simulink model "Subsystem2"  (R2020a)
settings: Solver=VariableStepAuto  StartTime=0.0  StopTime=10.0  RelTol=1e-3
settings Model: Creator=anjal  LastModifiedBy=anjal
settings DataIOCC: SaveOutput=off  SaveTime=off

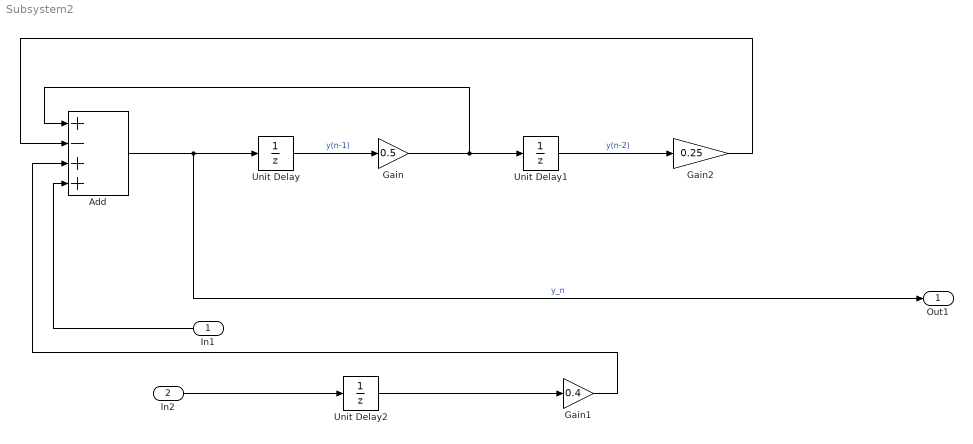
== system Subsystem2 ==
  In1 : Inport  OutDataTypeStr=double  PortDimensions=1  SampleTime=[0,1]
  In2 : Inport  Port=2  OutDataTypeStr=double  PortDimensions=1  SampleTime=[0,1]
  Add : Sum  Inputs=+-++
  Gain : Gain  Gain=0.5
  Gain1 : Gain  Gain=0.4
  Gain2 : Gain  Gain=0.25
  Unit Delay : UnitDelay  SampleTime=-1  HasFrameUpgradeWarning=on
  Unit Delay1 : UnitDelay  SampleTime=-1  HasFrameUpgradeWarning=on
  Unit Delay2 : UnitDelay  SampleTime=-1  HasFrameUpgradeWarning=on
  Out1 : Outport  OutDataTypeStr=double  PortDimensions=1  SampleTime=[0,1]
  wires:
  Add/1 -> Unit Delay/1, Out1/1  "y_n"
  Unit Delay/1 -> Gain/1  "y(n-1)"
  Unit Delay2/1 -> Gain1/1
  Gain/1 -> Add/1, Unit Delay1/1
  Unit Delay1/1 -> Gain2/1  "y(n-2)"
  Gain2/1 -> Add/2
  Gain1/1 -> Add/3
  In2/1 -> Unit Delay2/1
  In1/1 -> Add/4
